simulink model "cmdvel2gazebo"  (R2017a)
settings: Solver=FixedStepAuto  StartTime=0.0  StopTime=inf  FixedStep=0.02  RelTol=1e-3  EnableMultiTasking=on
libraries: robotlib x9
settings Model: Creator=sprinkle  LastModifiedBy=ece446
settings DataIOCC: LimitDataPoints=on
settings OptimizationCC: LifeSpan=Inf  MaxStackSize=64
settings DebuggingCC: AllowSymbolicDim=off  SFUnexpectedBacktrackingDiag=warning  SFNoUnconditionalDefaultTransitionDiag=warning  SFExecutionAtInitializationDiag=none
settings HardwareCC: ProdBitPerPointer=32  ProdBitPerSizeT=32  ProdBitPerPtrDiffT=32  ProdLargestAtomicFloat=None  ProdWordSize=32  ProdHWDeviceType=Custom Processor->Custom
settings ModelReferenceCC: PropagateSignalLabelsOutOfModel=off
settings SFSimCC: MATLABDynamicMemAlloc=off
settings RTWCC: SystemTargetFile=ert.tlc  HardwareBoard=Robot Operating System (ROS)  TLCOptions=-aInlineSetEventsForThisBaseRateFcn=TLC_FALSE -aSuppressMultiTaskScheduler=TLC_FALSE -aRateBasedStepFcn=0  TemplateMakefile=ert_default_tmf  Description=Embedded Coder  GenerateReport=on  Toolchain=Catkin  IncludeHyperlinkInReport=on  LaunchReport=on  TargetLang=C++  GenerateTraceInfo=on  GenerateTraceReport=on  GenerateTraceReportSl=on  GenerateTraceReportSf=on  GenerateTraceReportEml=on
settings CodeAppCC: ForceParamTrailComments=on  IgnoreCustomStorageClasses=off  OperatorAnnotations=on  SimulinkDataObjDesc=on  SFDataObjDesc=on  MATLABFcnDesc=on  InsertBlockDesc=on  MATLABSourceComments=on
settings ERTTargetCC: MultiwordLength=2048  SupportContinuousTime=on
settings ConfigComp: CovMetricSettings=dw  CovHtmlReporting=on  CovSaveCumulativeToWorkspaceVar=on  CovSaveSingleToWorkspaceVar=on  CovExternalEMLEnable=off

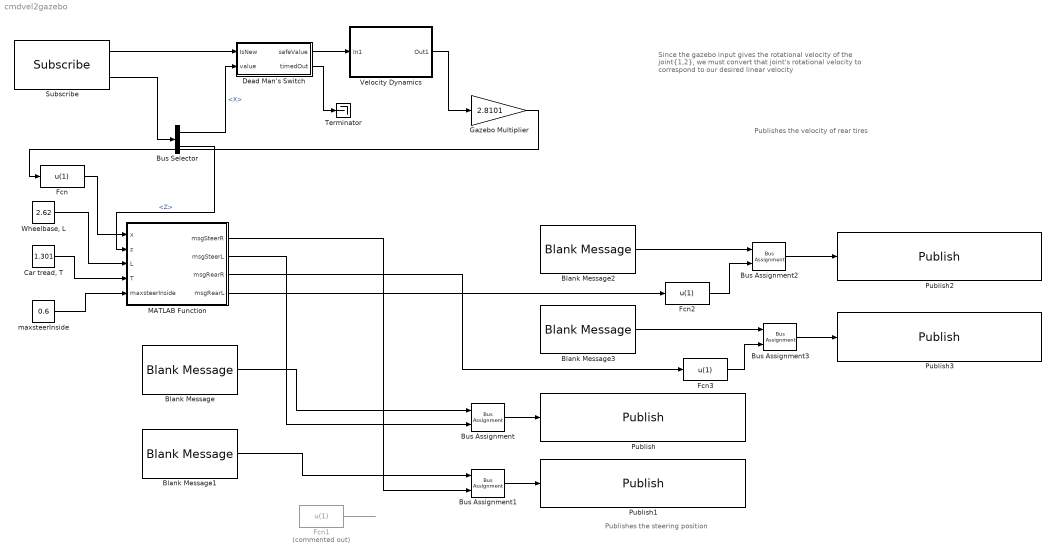
== system cmdvel2gazebo ==
  note: Since the gazebo input gives the rotational velocity of
      | the joint{1,2}, we must convert that joint's rotational velocity
      | to correspond to our desired linear velocity
  note: Publishes the steering position
  note: Publishes the velocity of rear tires
  Blank Message{,1..3} (4 alike) : robotlib/Blank Message  SourceLibraryInfo=This block requires Robotics System Toolbox  messageType=std_msgs/Float64  SampleTime=inf
      settings: SourceProductBaseCode=RO
  Bus Assignment{,1..3} (4 alike) : BusAssignment  AssignedSignals=Data
  Bus Selector : BusSelector  OutputSignals=Linear.X,Angular.Z
  "Car tread, T" : Constant  Value=1.301
  Dead Man's Switch : Subsystem  TreatAsAtomicUnit=on  mask{stepSize=0.01, timeout=0.2}
      mask prompts: stepSize "Simulation step size"; timeout "Timeout (in seconds)"
      mask help: Interprets whether a new message has been recently received, and if so permits the data in 'value' to be passed through. Otherwise, 0 is outputted from 'safeValue'
      mask Help: Interprets whether a new message has been recently received, and if so permits the data in 'value' to be passed through. Otherwise, 0 is outputted from 'safeValue'
  Fcn : Fcn  Expr=u(1)
  Fcn1 : Fcn  Commented=on  Expr=u(1)
  Fcn2 : Fcn  Expr=u(1)
  Fcn3 : Fcn  Expr=u(1)
  Gazebo Multiplier : Gain  Gain=2.8101
  MATLAB Function : MATLAB Function  TreatAsAtomicUnit=on
  Publish : robotlib/Publish  SourceLibraryInfo=This block requires Robotics System Toolbox  topicSource=Specify your own  topic=front_left_steering_position_controller/command  messageType=std_msgs/Float64  messageQueueLength=1
      settings: SourceProductBaseCode=RO
  Publish1 : robotlib/Publish  SourceLibraryInfo=This block requires Robotics System Toolbox  topicSource=Specify your own  topic=front_right_steering_position_controller/command  messageType=std_msgs/Float64  messageQueueLength=1
      settings: SourceProductBaseCode=RO
  Publish2 : robotlib/Publish  SourceLibraryInfo=This block requires Robotics System Toolbox  topicSource=Specify your own  topic=joint1_velocity_controller/command  messageType=std_msgs/Float64  messageQueueLength=1
      settings: SourceProductBaseCode=RO
  Publish3 : robotlib/Publish  SourceLibraryInfo=This block requires Robotics System Toolbox  topicSource=Specify your own  topic=joint2_velocity_controller/command  messageType=std_msgs/Float64  messageQueueLength=1
      settings: SourceProductBaseCode=RO
  Subscribe : robotlib/Subscribe  SourceLibraryInfo=This block requires Robotics System Toolbox  topicSource=Specify your own  topic=cmd_vel  messageType=geometry_msgs/Twist  sampleTime=-1  messageQueueLength=1
      settings: SourceProductBaseCode=RO
  Terminator : Terminator
  Velocity Dynamics : Subsystem
  "Wheelbase, L" : Constant  Value=2.62
  maxsteerInside : Constant  Value=0.6
  wires:
  Subscribe/2 -> Bus Selector/1
  Subscribe/1 -> Dead Man's Switch/1(IsNew)
  Blank Message/1 -> Bus Assignment/1
  Bus Assignment/1 -> Publish/1
  Blank Message1/1 -> Bus Assignment1/1
  Bus Assignment1/1 -> Publish1/1
  Blank Message2/1 -> Bus Assignment2/1
  Bus Assignment2/1 -> Publish2/1
  Blank Message3/1 -> Bus Assignment3/1
  Bus Assignment3/1 -> Publish3/1
  Velocity Dynamics/1(Out1) -> Gazebo Multiplier/1
  Fcn/1 -> MATLAB Function/1(x)
  Fcn1/1 -> ?
  Fcn2/1 -> Bus Assignment2/2
  Fcn3/1 -> Bus Assignment3/2
  Bus Selector/1 -> Dead Man's Switch/2(value)  "<X>"
  Dead Man's Switch/1(safeValue) -> Velocity Dynamics/1(In1)
  Dead Man's Switch/2(timedOut) -> Terminator/1
  maxsteerInside/1 -> MATLAB Function/5(maxsteerInside)
  "Wheelbase, L"/1 -> MATLAB Function/3(L)
  "Car tread, T"/1 -> MATLAB Function/4(T)
  Bus Selector/2 -> MATLAB Function/2(z)  "<Z>"
  MATLAB Function/1(msgSteerR) -> Bus Assignment1/2
  MATLAB Function/2(msgSteerL) -> Bus Assignment/2
  Gazebo Multiplier/1 -> Fcn/1
  MATLAB Function/4(msgRearL) -> Fcn2/1
  MATLAB Function/3(msgRearR) -> Fcn3/1

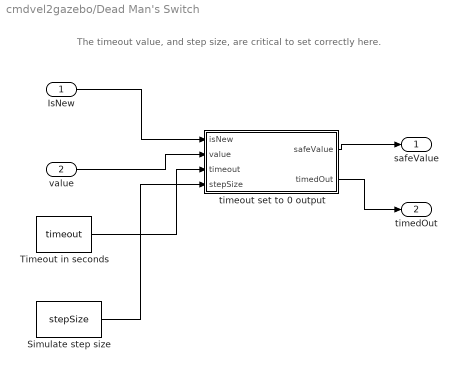
== system cmdvel2gazebo/Dead Man's Switch ==
  note: The timeout value, and step size, are critical to set correctly here.
  IsNew : Inport
  value : Inport  Port=2
  Simulate step size : Constant  Value=stepSize
  Timeout in seconds : Constant  Value=timeout
  timeout set to 0 output : MATLAB Function  TreatAsAtomicUnit=on
  safeValue : Outport  InitialOutput=[0]
  timedOut : Outport  Port=2  InitialOutput=[0]
  wires:
  IsNew/1 -> timeout set to 0 output/1(isNew)
  timeout set to 0 output/1(safeValue) -> safeValue/1
  value/1 -> timeout set to 0 output/2(value)
  Timeout in seconds/1 -> timeout set to 0 output/3(timeout)
  timeout set to 0 output/2(timedOut) -> timedOut/1
  Simulate step size/1 -> timeout set to 0 output/4(stepSize)

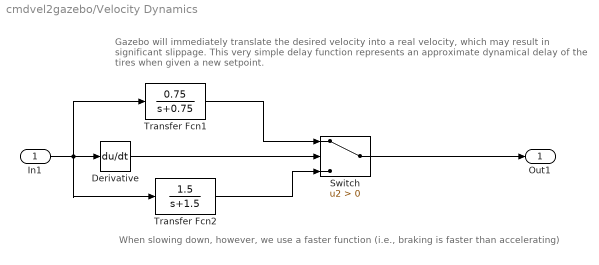
== system cmdvel2gazebo/Velocity Dynamics ==
  note: Gazebo will immediately translate the desired velocity into a real velocity, which may result in
      | significant slippage. This very simple delay function represents an approximate dynamical delay
      | of the tires when given a new setpoint.
  note: When slowing down, however, we use a faster function (i.e., braking is faster than accelerating)
  In1 : Inport
  Derivative : Derivative
  Switch : Switch  Criteria=u2 > Threshold
  Transfer Fcn1 : TransferFcn  Numerator=[0.75]  Denominator=[1 0.75]
  Transfer Fcn2 : TransferFcn  Numerator=[1.5]  Denominator=[1 1.5]
  Out1 : Outport
  wires:
  In1/1 -> Transfer Fcn1/1, Transfer Fcn2/1, Derivative/1
  Derivative/1 -> Switch/2
  Transfer Fcn1/1 -> Switch/1
  Switch/1 -> Out1/1
  Transfer Fcn2/1 -> Switch/3

== matlab function cmdvel2gazebo/MATLAB Function ==
  data: x input; z input; msgSteerR output; L input; T input; maxsteerInside input; msgSteerL output; msgRearR output; msgRearL output
function [msgSteerR, msgSteerL, msgRearR, msgRearL] = fcn(x, z, L, T, maxsteerInside)
%#codegen
rMax = L/tan(maxsteerInside);
rIdeal = rMax+(T/2.0);
maxsteer=atan2(L,rIdeal);

z = max(-maxsteer,min(maxsteer,z));
if( z ==0 )
    msgSteerL = z;
    msgSteerR = z;
    msgRearR  = x;
    msgRearL = x;
else
    r = L/abs(tan(z));
    rL = r-(sign(z)*(T/2.0));
    rR = r+(sign(z)*(T/2.0));
    msgRearR = x*rR/r;
    msgRearL = x*rL/r;
    
    msgSteerL = atan2(L,rL)*sign(z);
    msgSteerR = atan2(L,rR)*sign(z);

end

== matlab function cmdvel2gazebo/Dead Man's Switch/timeout set to 0 output ==
  data: isNew input; safeValue output; value input; timeout input; timedOut output; stepSize input
function [safeValue,timedOut] = fcn(isNew,value,timeout,stepSize)
%#codegen
persistent sinceLastMsg
timedOut=true;
if isempty(sinceLastMsg)
    sinceLastMsg=(timeout/stepSize)+1;
end

safeValue=0;
% if no new message
% after timeout, we output 0
if( isNew == true )
    sinceLastMsg = 0;
else
    sinceLastMsg = sinceLastMsg+1;
end

% Note: we require step size as an input here, and depend on our
% system being executed at a regular rate, or bad things will happen
if( sinceLastMsg < timeout/stepSize )
    timedOut = false;
end
    
if( timedOut == false )
    safeValue = value;
end
